simulink model "n5_feedback_linearization_LTI_controller"  (R2023b)
settings: Solver=VariableStepAuto  StartTime=0.0  StopTime=5  RelTol=1e-3
values from neighbouring files (symbols this model uses):
  dx_0 = [0;1;0;1]*0.01    [n0_collaborative_class_main.m]    (also in svc_robot.m = [0;1;0;1]*0.1)
  Kv_tilde = place(A_tilde, B_tilde, p_tilde)    [collaborative_class_main.m]    (also in n0_collaborative_class_main.m)
  u_bar = m*g*l*cos(x2_bar)    [collaborative_class_main.m]    (also in n0_collaborative_class_main.m; svc_robot.m)
libraries: cstblocks x1
settings Model: Creator=Kevin  LastModifiedBy=alexandraspertini

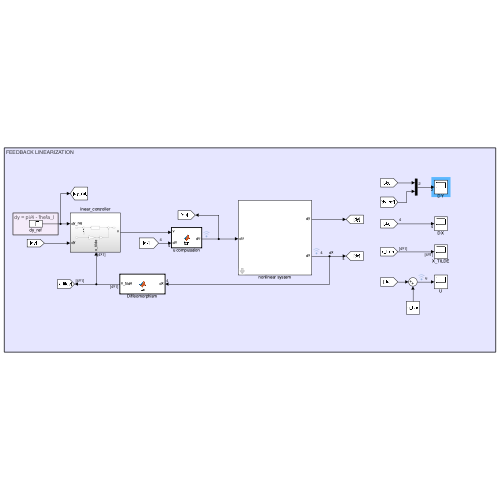
[thumbnail: Simulink's stored preview of the top-level diagram]
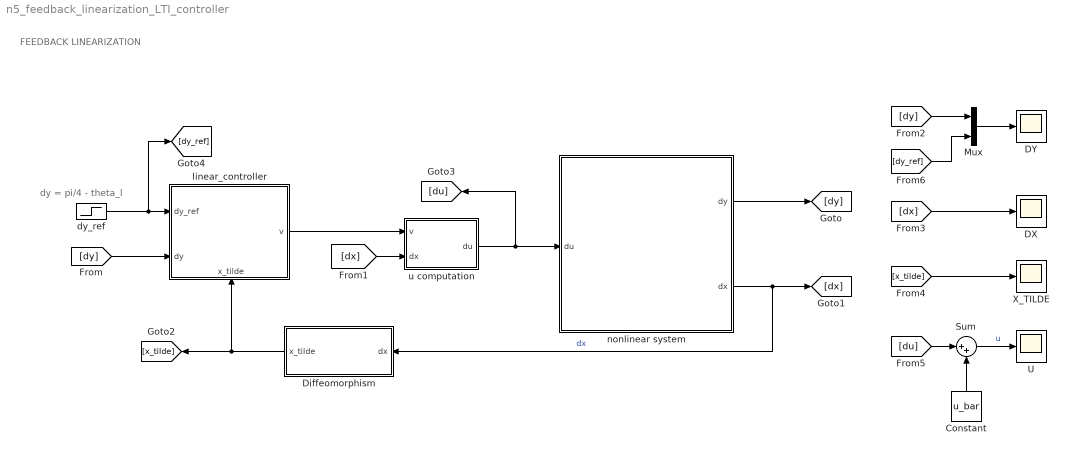
== system n5_feedback_linearization_LTI_controller ==
  note: dy = pi/4 - theta_l
  note: FEEDBACK LINEARIZATION
  Constant : Constant  Value=u_bar
  DX : Scope
  DY : Scope
  Diffeomorphism : MATLAB Function  TreatAsAtomicUnit=on
  Mux : Mux  Inputs=2
  Sum : Sum  Inputs=|++
  U : Scope
  X_TILDE : Scope
  dy_ref : Step  Time=1.5  SampleTime=0
  linear_controller : Subsystem
      settings: PortSchema="{\"entries\":[{\"content\":{\"sides\":[{\"content\":{\"connectorIds\":[\"In1\",\"In2\"]},\"type\":\"ConnectorPlacement.EquallySpacedRectSide\",\"uuid\":\"c2092a16-db5b-47d5-8a98-9be1c813ca90\"},{\"content\":{\"connectorIds\":[\"Out1\"],\"side\":\"RIGHT\"},\"type\":\"ConnectorPlacement.EquallySpacedRectSide\",\"uuid\":\"8bac7360-3a68-4504-9a33-81ae556d44dc\"},{\"content\":{\"side\":\"TOP\"},\"type\":\"ConnectorPlacement.EquallySpacedRectSide\",\"uuid\":\"a25b13c9-1d0d-47d6-baaf-c9e7bd37208a\"},{\"content\":{\"connectorIds\":[\"In3\"],\"side\":\"BOTTOM\"},\"type\":\"ConnectorPlacement.EquallySpacedRectSide\",\"uuid\":\"6ea912a5-9e35-4601-b2d1-80885da92b3f\"}]},\"type\":\"ConnectorPlacement.EquallySpacedConnector\",\"uuid\":\"2e31c0b4-3b1d-40f4-b6df-7c92d43c76f2\"}],\"packageUris\":[\"http://schema.mathworks.com/mf0/Connector/R2020b\"],\"version\":\"1.0\"}"
  nonlinear system : Subsystem  mask{dx_0=dx_0}
      mask prompts: dx_0 "initial condition"
  u computation : MATLAB Function  TreatAsAtomicUnit=on
  wires:
  nonlinear system/2(dx) -> [dx], Diffeomorphism/1(dx)  "dx"
  nonlinear system/1(dy) -> [dy]
  [dy] -> linear_controller/2(dy)
  dy_ref/1 -> [dy_ref], linear_controller/1(dy_ref)
  Constant/1 -> Sum/2
  Sum/1 -> U/1  "u"
  u computation/1(du) -> [du], nonlinear system/1(du)
  linear_controller/1(v) -> u computation/1(v)
  Diffeomorphism/1(x_tilde) -> [x_tilde], linear_controller/3(x_tilde)
  [dx] -> u computation/2(dx)
  [dx] -> DX/1
  [x_tilde] -> X_TILDE/1
  [du] -> Sum/1
  [dy] -> Mux/1
  Mux/1 -> DY/1
  [dy_ref] -> Mux/2

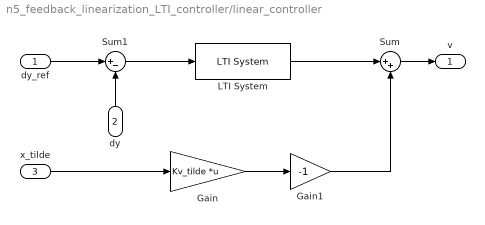
== system n5_feedback_linearization_LTI_controller/linear_controller ==
  dy_ref : Inport
  dy : Inport  Port=2
  x_tilde : Inport  Port=3
  Gain : Gain  Gain=Kv_tilde  Multiplication=Matrix(K*u) (u vector)
  Gain1 : Gain  Gain=-1
  LTI System : cstblocks/LTI System  sys=R_v  IC=[]  PadeOrder=0
  Sum : Sum  Inputs=|++
  Sum1 : Sum  Inputs=|+-
  v : Outport
  wires:
  Gain/1 -> Gain1/1
  x_tilde/1 -> Gain/1
  Gain1/1 -> Sum/2
  Sum/1 -> v/1
  dy/1 -> Sum1/2
  dy_ref/1 -> Sum1/1
  Sum1/1 -> LTI System/1
  LTI System/1 -> Sum/1

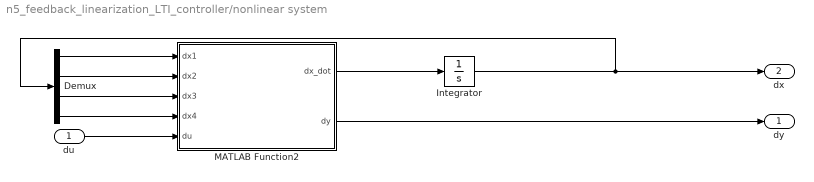
== system n5_feedback_linearization_LTI_controller/nonlinear system ==
  du : Inport
  Demux : Demux
  Integrator : Integrator  InitialCondition=[0;0;0;0]+ [0;1;0;1]*0.1
  MATLAB Function2 : MATLAB Function  TreatAsAtomicUnit=on
  dy : Outport
  dx : Outport  Port=2
  wires:
  Integrator/1 -> Demux/1, dx/1
  du/1 -> MATLAB Function2/5(du)
  MATLAB Function2/2(dy) -> dy/1
  MATLAB Function2/1(dx_dot) -> Integrator/1
  Demux/1 -> MATLAB Function2/1(dx1)
  Demux/2 -> MATLAB Function2/2(dx2)
  Demux/3 -> MATLAB Function2/3(dx3)
  Demux/4 -> MATLAB Function2/4(dx4)

== matlab function n5_feedback_linearization_LTI_controller/u computation ==
  data: v input; dx input; du output
function du  = fcn(v, dx)

%v = 0;
k = 0.8;
Jm = 4e-4;
Jl= 4e-4;
Bm = 0.015;
m = 0.3;
l = 0.3;
g = 9.81;

x1_bar = 0;
x2_bar = pi/4;
x3_bar = 0;
x4_bar = m*g*l*cos(x2_bar)/k + x2_bar;
u_bar= m*g*l*cos(x2_bar);

x1 = dx(1)+x1_bar;
x2 = dx(2)+x2_bar;
x3 = dx(3)+x3_bar;
x4 = dx(4)+x4_bar;

% HARDCODED
%u = Jl*Jm/k* (   -v+k^2/Jl^2*(x4-x2)     +   m*g*l*k/Jl^2*(sin(x2)*x2-cos(x2)-sin(x2)*x4)   -    m*g*l/Jl*cos(x2)*x1^2    +   m^2*g^2*l^2/(-Jl^2)*sin(x2)*cos(x2)    +   k^2/(Jl*Jm)*(x2-x4)     +   k*Bm/(Jl*Jm)*x3);

% from MATLAB INVERSION
 u = -(Jl*Jm*((g*l*m*cos(x2)*x1^2)/Jl + v - (k*((Bm*x3)/Jm - (k*x2)/Jm + (k*x4)/Jm))/Jl + (k*((k*x2)/Jl - (k*x4)/Jl + (g*l*m*cos(x2))/Jl))/Jl - (g*l*m*sin(x2)*((k*x2)/Jl - (k*x4)/Jl + (g*l*m*cos(x2))/Jl))/Jl))/k;
du = u - u_bar;

== matlab function n5_feedback_linearization_LTI_controller/nonlinear system/MATLAB Function2 ==
  data: dx1 input; dx2 input; dx3 input; dx4 input; du input; dx_dot output; dy output
function [dx_dot, dy]  = fcn(dx1,dx2,dx3,dx4, du)

k = 0.8;
Jm = 4e-4;
Jl= 4e-4;
Bm = 0.015;
Bl = 0;
m = 0.3;
l = 0.3;
g = 9.81;
x1_bar = 0;
x2_bar = pi/4;
x3_bar = 0;
x4_bar = m*g*l*cos(x2_bar)/k + x2_bar;
u_bar= m*g*l*cos(x2_bar);


dx1_dot = -k/Jl*(dx2+x2_bar)-m*g*l/Jl*(cos(dx2+x2_bar))+k/Jl*(dx4+x4_bar);
dx2_dot = dx1+x1_bar;
dx3_dot = k/Jm*(dx2+x2_bar)-Bm/Jm*(dx3+x3_bar)-k/Jm*(dx4+x4_bar)+1/Jm*(du+u_bar);
dx4_dot = dx3+x3_bar;
dy = pi/4 - (dx2+x2_bar);

dx_dot = zeros(1,4);
dx_dot(1) = dx1_dot;
dx_dot(2) = dx2_dot;
dx_dot(3) = dx3_dot;
dx_dot(4) = dx4_dot;

== matlab function n5_feedback_linearization_LTI_controller/Diffeomorphism ==
  data: dx input; x_tilde output
function x_tilde  = fcn(dx)

dx1 = dx(1);
dx2 = dx(2);
dx3 = dx(3);
dx4 = dx(4);
k = 0.8;
Jm = 4e-4;
Jl= 4e-4;
Bm = 0.015;
Bl = 0;
m = 0.3;
l = 0.3;
g = 9.81;

x1_tilde = -dx2;
x2_tilde = -dx1;
x3_tilde = (k*(pi/4 + dx2))/Jl - (k*(dx4 + sqrt(2)/2*m*g*l/k+pi/4))/Jl + (g*l*m*cos(pi/4 + dx2))/Jl;
x4_tilde = (k*dx1)/Jl - (k*dx3)/Jl - (g*l*m*sin(pi/4 + dx2)*dx1)/Jl;

x_tilde = zeros(length(dx),1);
x_tilde(1) = x1_tilde;
x_tilde(2) = x2_tilde;
x_tilde(3) = x3_tilde;
x_tilde(4) = x4_tilde;
